simulink model "odporny_uklad_regulacji"  (R2024b)
settings: Solver=VariableStepAuto  StartTime=0.0  StopTime=100  MaxStep=0.01  RelTol=1e-3
values from neighbouring files (symbols this model uses):
  l = 1    [dane.m]
  m = [8 1]    [dane.m]
  Ts = 1    [dane.m]
undefined symbols (not defined in the file or in its folder): dspblkCoreblockFVToolHelper, gcbh
settings Model: Creator=rrost  LastModifiedBy=marci

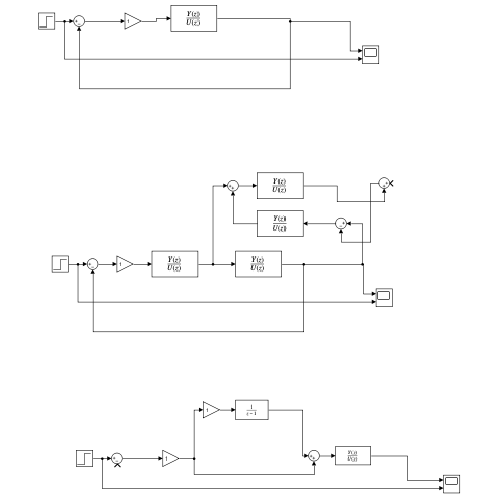
[thumbnail: Simulink's stored preview of the top-level diagram]
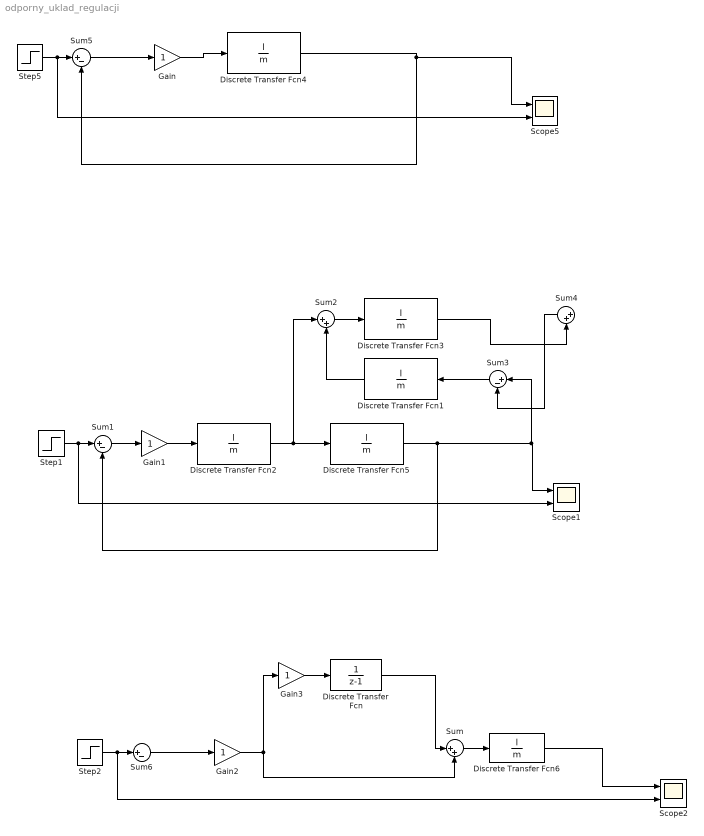
== system odporny_uklad_regulacji ==
  Discrete Transfer Fcn : DiscreteTransferFcn  LoadFcn=dspblkCoreblockFVToolHelper(gcbh,'load');  Denominator=[1 -1]
      settings: CopyFcn=dspblkCoreblockFVToolHelper(gcbh,'copy');  DeleteFcn=dspblkCoreblockFVToolHelper(gcbh,'close');  ModelCloseFcn=dspblkCoreblockFVToolHelper(gcbh,'close');  PreSaveFcn=dspblkCoreblockFVToolHelper(gcbh,'presave');  PostSaveFcn=dspblkCoreblockFVToolHelper(gcbh,'postsave');  CloseFcn=dspblkCoreblockFVToolHelper(gcbh,'close');
  Discrete Transfer Fcn{1..6} (6 alike) : DiscreteTransferFcn  LoadFcn=dspblkCoreblockFVToolHelper(gcbh,'load');  Numerator=l  Denominator=m  SampleTime=Ts
      settings: CopyFcn=dspblkCoreblockFVToolHelper(gcbh,'copy');  DeleteFcn=dspblkCoreblockFVToolHelper(gcbh,'close');  ModelCloseFcn=dspblkCoreblockFVToolHelper(gcbh,'close');  PreSaveFcn=dspblkCoreblockFVToolHelper(gcbh,'presave');  PostSaveFcn=dspblkCoreblockFVToolHelper(gcbh,'postsave');  CloseFcn=dspblkCoreblockFVToolHelper(gcbh,'close');
  Gain{,1..3} (4 alike) : Gain
  Scope1 : Scope  NumInputPorts=2
  Scope2 : Scope  NumInputPorts=2
  Scope5 : Scope  NumInputPorts=2
  Step1 : Step  SampleTime=1
  Step2 : Step  SampleTime=1
  Step5 : Step  SampleTime=1
  Sum : Sum  Inputs=|++
  Sum{1,3,5..6} (4 alike) : Sum  Inputs=|+-
  Sum2 : Sum  Inputs=|++
  Sum4 : Sum  Inputs=|++
  wires:
  Discrete Transfer Fcn4/1 -> Scope5/1, Sum5/2
  Step5/1 -> Scope5/2, Sum5/1
  Sum5/1 -> Gain/1
  Gain/1 -> Discrete Transfer Fcn4/1
  Step1/1 -> Scope1/2, Sum1/1
  Discrete Transfer Fcn2/1 -> Sum2/1, Discrete Transfer Fcn5/1
  Sum1/1 -> Gain1/1
  Gain1/1 -> Discrete Transfer Fcn2/1
  Sum2/1 -> Discrete Transfer Fcn3/1
  Discrete Transfer Fcn5/1 -> Sum3/1, Scope1/1, Sum1/2
  Sum3/1 -> Discrete Transfer Fcn1/1
  Sum4/1 -> Sum3/2
  Discrete Transfer Fcn1/1 -> Sum2/2
  Step2/1 -> Scope2/2, Sum6/1
  Sum6/1 -> Gain2/1
  Gain2/1 -> Sum/2, Gain3/1
  Discrete Transfer Fcn/1 -> Sum/1
  Sum/1 -> Discrete Transfer Fcn6/1
  Gain3/1 -> Discrete Transfer Fcn/1
  Discrete Transfer Fcn6/1 -> Scope2/1
  Discrete Transfer Fcn3/1 -> Sum4/2
